simulink model "swerve_4wd_generic_sim"  (R2022b)
settings: Solver=VariableStepAuto  StartTime=0.0  StopTime=inf  RelTol=1e-3  AbsTol=1e-3  EnableMultiTasking=on
PreLoadFcn:
  | R = 0.106 / 2.0; % [m] wheel radius
  | wheel_1_loc = [-0.2; 0.2];
  | wheel_2_loc = [0.2; 0.2];
  | wheel_3_loc = [-0.2; -0.2];
  | wheel_4_loc = [0.2; -0.2];
InitFcn:
  | R = 0.106 / 2.0; % [m] wheel radius
  | wheel_1_loc = [-0.2; 0.2];
  | wheel_2_loc = [0.2; 0.2];
  | wheel_3_loc = [-0.2; -0.2];
  | wheel_4_loc = [0.2; -0.2];
undefined symbols (not defined in the file): X, Y, Z
libraries: sm_lib x43, nesl_utility x17, dspsigops x2
(part 2 of 2)

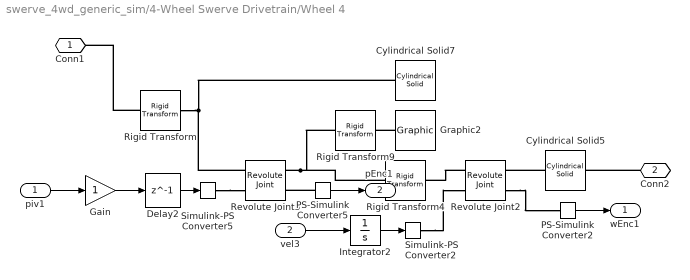
== system swerve_4wd_generic_sim/4-Wheel Swerve Drivetrain/Wheel 4 ==
  piv1 : Inport
  vel3 : Inport  Port=2
  Cylindrical Solid5 : sm_lib/Body Elements/Cylindrical Solid  GraphicAmbientColor=[0.15 0.15 0.15 1.0]  BasedOnType=Density  CenterOfMass=[0 0 0]  CenterOfMassUnits=m  GraphicDiffuseColor=[0.6 0.2 1.0]  CylinderLength=0.04  CylinderLengthUnits=m  CylinderRadius=0.106/2  CylinderRadiusUnits=m  Density=1000  DensityUnits=kg/m^3  DoExposeReferenceFrame=on  GraphicEmissiveColor=[0.0 0.0 0.0 1.0]  ExportEntireGeometry=on  SerializedFrames=<Frames/>  MarkerShape=Sphere  MarkerSize=10  GraphicType=FromGeometry  InertiaType=CalculateFromGeometry  Mass=1  MassUnits=kg  MomentsOfInertia=[1 1 1]  MomentsOfInertiaUnits=kg*m^2  GraphicOpacity=1.0  ProductsOfInertia=[0 0 0]  ProductsOfInertiaUnits=kg*m^2  GraphicShininess=75  GraphicSpecularColor=[0.5 0.5 0.5 1.0]  GraphicVisPropType=SimpleVisualProperties
  Cylindrical Solid7 : sm_lib/Body Elements/Cylindrical Solid  GraphicAmbientColor=[0.15 0.15 0.15 1.0]  BasedOnType=Density  CenterOfMass=[0 0 0]  CenterOfMassUnits=m  GraphicDiffuseColor=[0.0 0.6 0.4]  CylinderLength=0.04  CylinderLengthUnits=m  CylinderRadius=0.04  CylinderRadiusUnits=m  Density=1000  DensityUnits=kg/m^3  DoExposeReferenceFrame=on  GraphicEmissiveColor=[0.0 0.0 0.0 1.0]  ExportEntireGeometry=off  SerializedFrames=<Frames/>  MarkerShape=Sphere  MarkerSize=10  GraphicType=FromGeometry  InertiaType=CalculateFromGeometry  Mass=1  MassUnits=kg  MomentsOfInertia=[1 1 1]  MomentsOfInertiaUnits=kg*m^2  GraphicOpacity=0.3  ProductsOfInertia=[0 0 0]  ProductsOfInertiaUnits=kg*m^2  GraphicShininess=75  GraphicSpecularColor=[0.5 0.5 0.5 1.0]  GraphicVisPropType=SimpleVisualProperties
  Delay2 : Delay  DelayLength=1  InitialCondition=0
  Gain : Gain
  Graphic2 : sm_lib/Body Elements/Graphic  GraphicType=Marker  MarkerShape=Sphere  MarkerSize=10  GraphicVisPropType=SimpleVisualProperties  GraphicDiffuseColor=[1 0.5 0.5]  GraphicSpecularColor=[0.5 0.5 0.5 1.0]  GraphicAmbientColor=[0.15 0.15 0.15 1.0]  GraphicEmissiveColor=[0.0 0.0 0.0 1.0]  GraphicShininess=75  GraphicOpacity=1.0
  Integrator2 : Integrator
  PS-Simulink Converter2 : nesl_utility/PS-Simulink Converter  PhysicalDomain=network_engine_domain  SubClassName=ps_output  LeftPortType=input  RightPortType=output  PseudoPeriodic=off  Frequencies=[]  VectorFormat=1-D array  Unit=inherit  AffineConversion=off
  PS-Simulink Converter5 : nesl_utility/PS-Simulink Converter  PhysicalDomain=network_engine_domain  SubClassName=ps_output  LeftPortType=input  RightPortType=output  PseudoPeriodic=off  Frequencies=[]  VectorFormat=1-D array  Unit=inherit  AffineConversion=off
  Revolute Joint2 : sm_lib/Joints/Revolute Joint  JointMode=Normal  SenseConstraintForce=off  SenseConstraintForceX=off  SenseConstraintForceY=off  SenseConstraintForceZ=off  SenseConstraintTorque=off  SenseConstraintTorqueX=off  SenseConstraintTorqueY=off  SenseConstraintTorqueZ=off  SenseTotalForce=off  SenseTotalForceX=off  SenseTotalForceY=off  SenseTotalForceZ=off  SenseTotalTorque=off  SenseTotalTorqueX=off  SenseTotalTorqueY=off  SenseTotalTorqueZ=off  CompositeWrenchDir=FollowerOnBase  CompositeWrenchFrame=BaseFrame  EquilibriumPosition=0  EquilibriumPositionUnits=deg  SpringStiffness=0  SpringStiffnessUnits=N*m/deg  DampingCoefficient=0  DampingCoefficientUnits=N*m/(deg/s)  TorqueActuationMode=ComputedTorque  MotionActuationMode=InputMotion  SensePosition=on  SenseVelocity=off  SenseAcceleration=off  SenseTorqueForce=off  SenseLowerLimitTorqueForce=off  SenseUpperLimitTorqueForce=off  LowerLimitSpecify=off  LowerLimitBound=-90  LowerLimitBoundUnits=deg  LowerLimitStiffness=1e4  LowerLimitStiffnessUnits=N*m/deg  LowerLimitDamping=10  LowerLimitDampingUnits=N*m/(deg/s)  LowerLimitTransitionRegionWidth=0.1  LowerLimitTransitionRegionWidthUnits=deg  UpperLimitSpecify=off  UpperLimitBound=90  UpperLimitBoundUnits=deg  UpperLimitStiffness=1e4  UpperLimitStiffnessUnits=N*m/deg  UpperLimitDamping=10  UpperLimitDampingUnits=N*m/(deg/s)  UpperLimitTransitionRegionWidth=0.1  UpperLimitTransitionRegionWidthUnits=deg  PositionTargetSpecify=off  PositionTargetPriority=High  PositionTargetValue=0  PositionTargetValueUnits=deg  VelocityTargetSpecify=off  VelocityTargetPriority=High  VelocityTargetValue=0  VelocityTargetValueUnits=deg/s
  Revolute Joint5 : sm_lib/Joints/Revolute Joint  JointMode=Normal  SenseConstraintForce=off  SenseConstraintForceX=off  SenseConstraintForceY=off  SenseConstraintForceZ=off  SenseConstraintTorque=off  SenseConstraintTorqueX=off  SenseConstraintTorqueY=off  SenseConstraintTorqueZ=off  SenseTotalForce=off  SenseTotalForceX=off  SenseTotalForceY=off  SenseTotalForceZ=off  SenseTotalTorque=off  SenseTotalTorqueX=off  SenseTotalTorqueY=off  SenseTotalTorqueZ=off  CompositeWrenchDir=FollowerOnBase  CompositeWrenchFrame=BaseFrame  EquilibriumPosition=0  EquilibriumPositionUnits=deg  SpringStiffness=0  SpringStiffnessUnits=N*m/deg  DampingCoefficient=0  DampingCoefficientUnits=N*m/(deg/s)  TorqueActuationMode=ComputedTorque  MotionActuationMode=InputMotion  SensePosition=on  SenseVelocity=off  SenseAcceleration=off  SenseTorqueForce=off  SenseLowerLimitTorqueForce=off  SenseUpperLimitTorqueForce=off  LowerLimitSpecify=off  LowerLimitBound=-90  LowerLimitBoundUnits=deg  LowerLimitStiffness=1e4  LowerLimitStiffnessUnits=N*m/deg  LowerLimitDamping=10  LowerLimitDampingUnits=N*m/(deg/s)  LowerLimitTransitionRegionWidth=0.1  LowerLimitTransitionRegionWidthUnits=deg  UpperLimitSpecify=off  UpperLimitBound=90  UpperLimitBoundUnits=deg  UpperLimitStiffness=1e4  UpperLimitStiffnessUnits=N*m/deg  UpperLimitDamping=10  UpperLimitDampingUnits=N*m/(deg/s)  UpperLimitTransitionRegionWidth=0.1  UpperLimitTransitionRegionWidthUnits=deg  PositionTargetSpecify=off  PositionTargetPriority=High  PositionTargetValue=0  PositionTargetValueUnits=deg  VelocityTargetSpecify=off  VelocityTargetPriority=High  VelocityTargetValue=0  VelocityTargetValueUnits=deg/s
  Rigid Transform : sm_lib/Frames and Transforms/Rigid Transform  TranslationMethod=Cartesian  TranslationStandardOffset=0  TranslationLengthUnit=m  TranslationStandardAxis=+Z  TranslationCartesianOffset=[wheel_4_loc' 0]  TranslationROffset=0  TranslationROffsetUnits=m  TranslationZOffset=0  TranslationZOffsetUnits=m  TranslationThetaOffset=0  TranslationThetaOffsetUnits=deg  RotationMethod=None  RotationAngleUnits=deg  RotationStandardAxis=+Z  RotationAngle=0.0  RotationArbitraryAxis=[0 0 1]  FollAlignAxisA=+X  BaseAlignAxisA=+Y  FollAlignAxisB=+Y  BaseAlignAxisB=+Z  RotationSequenceAxes=FollowerAxes  RotationSequence=XYX  RotationSequenceAngles=[0 0 0]  RotationSequenceAnglesUnits=deg  RotationMatrix=[1 0 0; 0 1 0; 0 0 1]  Quaternion=[1 0 0 0]
  Rigid Transform4 : sm_lib/Frames and Transforms/Rigid Transform  TranslationMethod=Cartesian  TranslationStandardOffset=0  TranslationLengthUnit=m  TranslationStandardAxis=+Z  TranslationCartesianOffset=[0 0 -R-0.02]  TranslationROffset=0  TranslationROffsetUnits=m  TranslationZOffset=0  TranslationZOffsetUnits=m  TranslationThetaOffset=0  TranslationThetaOffsetUnits=deg  RotationMethod=StandardAxis  RotationAngleUnits=deg  RotationStandardAxis=+X  RotationAngle=90  RotationArbitraryAxis=[0 0 1]  FollAlignAxisA=+X  BaseAlignAxisA=+Y  FollAlignAxisB=+Y  BaseAlignAxisB=+Z  RotationSequenceAxes=FollowerAxes  RotationSequence=XYX  RotationSequenceAngles=[0 0 0]  RotationSequenceAnglesUnits=deg  RotationMatrix=[1 0 0; 0 1 0; 0 0 1]  Quaternion=[1 0 0 0]
  Rigid Transform9 : sm_lib/Frames and Transforms/Rigid Transform  TranslationMethod=Cartesian  TranslationStandardOffset=0  TranslationLengthUnit=m  TranslationStandardAxis=+Z  TranslationCartesianOffset=[0.1 0 0]  TranslationROffset=0  TranslationROffsetUnits=m  TranslationZOffset=0  TranslationZOffsetUnits=m  TranslationThetaOffset=0  TranslationThetaOffsetUnits=deg  RotationMethod=None  RotationAngleUnits=deg  RotationStandardAxis=+X  RotationAngle=90  RotationArbitraryAxis=[0 0 1]  FollAlignAxisA=+X  BaseAlignAxisA=+Y  FollAlignAxisB=+Y  BaseAlignAxisB=+Z  RotationSequenceAxes=FollowerAxes  RotationSequence=XYX  RotationSequenceAngles=[0 0 0]  RotationSequenceAnglesUnits=deg  RotationMatrix=[1 0 0; 0 1 0; 0 0 1]  Quaternion=[1 0 0 0]
  Simulink-PS Converter2 : nesl_utility/Simulink-PS Converter  PhysicalDomain=network_engine_domain  SubClassName=ps_input  LeftPortType=input  RightPortType=output  PseudoPeriodic=off  Frequencies=[]  NoiseDistribution=none  NoiseParameters=[]  Unit=1  AffineConversion=off  FilteringAndDerivatives=filter  SimscapeFilterOrder=2  InputFilterTimeConstant=0.001  UdotUserProvided=0
  Simulink-PS Converter5 : nesl_utility/Simulink-PS Converter  PhysicalDomain=network_engine_domain  SubClassName=ps_input  LeftPortType=input  RightPortType=output  PseudoPeriodic=off  Frequencies=[]  NoiseDistribution=none  NoiseParameters=[]  Unit=1  AffineConversion=off  FilteringAndDerivatives=filter  SimscapeFilterOrder=2  InputFilterTimeConstant=0.001  UdotUserProvided=0
  Conn1 : PMIOPort  Side=Left
  Conn2 : PMIOPort  Port=2  Side=Right
  wEnc1 : Outport
  pEnc1 : Outport  Port=2
  wires:
  Gain/1 -> Delay2/1
  piv1/1 -> Gain/1
  PS-Simulink Converter2/1 -> wEnc1/1
  vel3/1 -> Integrator2/1
  PS-Simulink Converter5/1 -> pEnc1/1
  Integrator2/1 -> Simulink-PS Converter2/1
  Delay2/1 -> Simulink-PS Converter5/1
  connections:
  Revolute Joint5/RConn1 -- Rigid Transform4/LConn1 -- Rigid Transform9/LConn1
  Conn2/RConn1 -- Cylindrical Solid5/LConn1
  Graphic2/RConn1 -- Rigid Transform9/RConn1
  Cylindrical Solid5/RConn1 -- Revolute Joint2/RConn1
  Revolute Joint2/RConn2 -- PS-Simulink Converter2/LConn1
  Rigid Transform/RConn1 -- Revolute Joint5/LConn1 -- Cylindrical Solid7/RConn1
  Simulink-PS Converter5/RConn1 -- Revolute Joint5/LConn2
  PS-Simulink Converter5/LConn1 -- Revolute Joint5/RConn2
  Revolute Joint2/LConn1 -- Rigid Transform4/RConn1
  Simulink-PS Converter2/RConn1 -- Revolute Joint2/LConn2
  Rigid Transform/LConn1 -- Conn1/RConn1

== matlab function swerve_4wd_generic_sim/Low Level Control/vel_local_ref_to_wheel_vel ==
  data: vel_local_ref input; pivots_rad output; wheel_vels_rad_s output
function [pivots_rad, wheel_vels_rad_s] = swerve_kinematics(vel_local_ref)
pivots_rad = zeros(4,1);
wheel_vels_rad_s = zeros(4,1);

R = 0.106 / 2.0; % [m] wheel radius

% Wheel definitions
wheel_1_loc = [-0.2; 0.2];
wheel_1_arm = sqrt(wheel_1_loc(1).^2 + wheel_1_loc(2).^2);
wheel_1_angle = atan2(wheel_1_loc(2), wheel_1_loc(1)) + pi/2;

wheel_2_loc = [0.2; 0.2];
wheel_2_arm = sqrt(wheel_2_loc(1).^2 + wheel_2_loc(2).^2);
wheel_2_angle = atan2(wheel_2_loc(2), wheel_2_loc(1)) + pi/2;

wheel_3_loc = [-0.2; -0.2];
wheel_3_arm = sqrt(wheel_3_loc(1).^2 + wheel_3_loc(2).^2);
wheel_3_angle = atan2(wheel_3_loc(2), wheel_3_loc(1)) + pi/2;

wheel_4_loc = [0.2; -0.2];
wheel_4_arm = sqrt(wheel_4_loc(1).^2 + wheel_4_loc(2).^2);
wheel_4_angle = atan2(wheel_4_loc(2), wheel_4_loc(1)) + pi/2;

% Linear velocity components
vel_x = vel_local_ref(1);
vel_y = vel_local_ref(2);

wheel_1_vel = [vel_x; vel_y];
wheel_2_vel = [vel_x; vel_y];
wheel_3_vel = [vel_x; vel_y];
wheel_4_vel = [vel_x; vel_y];

% Rotational velocity components
vel_phi = vel_local_ref(3);

wheel_1_rot_vel = vel_phi*wheel_1_arm;
wheel_1_vel = wheel_1_vel + [cos(wheel_1_angle)* wheel_1_rot_vel; sin(wheel_1_angle)*wheel_1_rot_vel];

wheel_2_rot_vel = vel_phi*wheel_2_arm;
wheel_2_vel = wheel_2_vel + [cos(wheel_2_angle)* wheel_2_rot_vel; sin(wheel_2_angle)*wheel_2_rot_vel];

wheel_3_rot_vel = vel_phi*wheel_3_arm;
wheel_3_vel = wheel_3_vel + [cos(wheel_3_angle)* wheel_3_rot_vel; sin(wheel_3_angle)*wheel_3_rot_vel];

wheel_4_rot_vel = vel_phi*wheel_4_arm;
wheel_4_vel = wheel_4_vel + [cos(wheel_4_angle)* wheel_4_rot_vel; sin(wheel_4_angle)*wheel_4_rot_vel];

% Get results
pivots_rad(1) = atan2(wheel_1_vel(2), wheel_1_vel(1));
pivots_rad(2) = atan2(wheel_2_vel(2), wheel_2_vel(1));
pivots_rad(3) = atan2(wheel_3_vel(2), wheel_3_vel(1));
pivots_rad(4) = atan2(wheel_4_vel(2), wheel_4_vel(1));

wheel_vels_rad_s(1) = sqrt(wheel_1_vel(1).^2 + wheel_1_vel(2).^2) / R;
wheel_vels_rad_s(2) = sqrt(wheel_2_vel(1).^2 + wheel_2_vel(2).^2) / R;
wheel_vels_rad_s(3) = sqrt(wheel_3_vel(1).^2 + wheel_3_vel(2).^2) / R;
wheel_vels_rad_s(4) = sqrt(wheel_4_vel(1).^2 + wheel_4_vel(2).^2) / R;
